simulink model "Preisach_1"  (R2015a)
settings: Solver=ode3  StartTime=0.0  StopTime=10.0  FixedStep=0.001  RelTol=1e-3
settings Model: Creator=spikelucky  LastModifiedBy=kr2112
settings DebuggingCC: UnderspecifiedInitializationDetection=Classic  MergeDetectMultiDrivingBlocksExec=none  SolverPrmCheckMsg=warning  StateNameClashWarn=warning

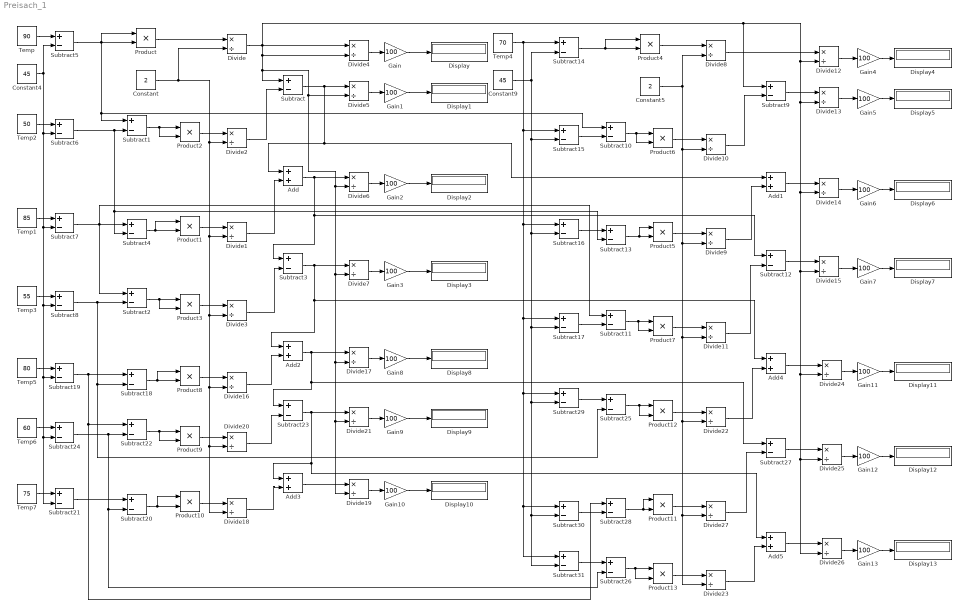
== system Preisach_1 ==
  Add{,1..5} (6 alike) : Sum
  Constant : Constant  Value=2
  Constant4 : Constant  Value=45
  Constant5 : Constant  Value=2
  Constant9 : Constant  Value=45
  Display{,1..13} (14 alike) : Display
  Divide{,1..27} (28 alike) : Product  Inputs=*/
  Gain{,1..13} (14 alike) : Gain  Gain=100
  Product{,1..13} (14 alike) : Product
  Subtract{,1..31} (32 alike) : Sum  Inputs=+-
  Temp : Constant  Value=90
  Temp1 : Constant  Value=85
  Temp2 : Constant  Value=50
  Temp3 : Constant  Value=55
  Temp4 : Constant  Value=70
  Temp5 : Constant  Value=80
  Temp6 : Constant  Value=60
  Temp7 : Constant  Value=75
  wires:
  Temp/1 -> Subtract5/1
  Product/1 -> Divide/1
  Product2/1 -> Divide2/1
  Divide2/1 -> Subtract/2
  Subtract1/1 -> Product2/2, Product2/1
  Product1/1 -> Divide1/1
  Divide1/1 -> Add/2
  Add/1 -> Divide6/1, Subtract3/1, Subtract12/1
  Product3/1 -> Divide3/1
  Subtract2/1 -> Product3/2, Product3/1
  Divide3/1 -> Subtract3/2
  Subtract4/1 -> Product1/2, Product1/1
  Divide4/1 -> Gain/1
  Gain/1 -> Display/1
  Gain1/1 -> Display1/1
  Divide5/1 -> Gain1/1
  Divide6/1 -> Gain2/1
  Gain2/1 -> Display2/1
  Divide7/1 -> Gain3/1
  Gain3/1 -> Display3/1
  Subtract3/1 -> Add4/1, Add2/1, Divide7/1
  Constant4/1 -> Subtract21/2, Subtract24/2, Subtract19/2, Subtract8/2, Subtract7/2, Subtract6/2, Subtract5/2
  Subtract5/1 -> Subtract10/1, Subtract1/1, Product/1, Product/2
  Subtract6/1 -> Subtract13/2, Subtract4/2, Subtract1/2
  Temp2/1 -> Subtract6/1
  Subtract7/1 -> Subtract2/1, Subtract11/1, Subtract4/1
  Temp1/1 -> Subtract7/1
  Subtract8/1 -> Subtract25/2, Subtract18/2, Subtract2/2
  Temp3/1 -> Subtract8/1
  Product4/1 -> Divide8/1
  Product6/1 -> Divide10/1
  Divide8/1 -> Divide12/1
  Divide10/1 -> Subtract9/2
  Subtract9/1 -> Divide13/1
  Subtract10/1 -> Product6/1, Product6/2
  Product5/1 -> Divide9/1
  Divide9/1 -> Add1/2
  Add1/1 -> Divide14/1
  Product7/1 -> Divide11/1
  Subtract11/1 -> Product7/2, Product7/1
  Divide11/1 -> Subtract12/2
  Subtract13/1 -> Product5/2, Product5/1
  Divide12/1 -> Gain4/1
  Gain4/1 -> Display4/1
  Gain5/1 -> Display5/1
  Divide13/1 -> Gain5/1
  Divide14/1 -> Gain6/1
  Gain6/1 -> Display6/1
  Divide15/1 -> Gain7/1
  Gain7/1 -> Display7/1
  Subtract12/1 -> Divide15/1
  Subtract14/1 -> Product4/1, Product4/2
  Subtract15/1 -> Subtract10/2
  Subtract16/1 -> Subtract13/1
  Subtract17/1 -> Subtract11/2
  Product8/1 -> Divide16/1
  Subtract18/1 -> Product8/2, Product8/1
  Subtract19/1 -> Subtract28/1, Subtract22/1, Subtract18/1
  Temp5/1 -> Subtract19/1
  Divide17/1 -> Gain8/1
  Gain8/1 -> Display8/1
  Divide16/1 -> Add2/2
  Product9/1 -> Divide20/1
  Subtract22/1 -> Product9/2, Product9/1
  Divide20/1 -> Subtract23/2
  Divide21/1 -> Gain9/1
  Gain9/1 -> Display9/1
  Subtract23/1 -> Add5/1, Add3/1, Divide21/1
  Subtract24/1 -> Subtract26/2, Subtract20/2, Subtract22/2
  Temp6/1 -> Subtract24/1
  Constant/1 -> Divide18/2, Divide20/2, Divide16/2, Divide3/2, Divide1/2, Divide2/2, Divide/2
  Product10/1 -> Divide18/1
  Subtract20/1 -> Product10/2, Product10/1
  Subtract21/1 -> Subtract20/1
  Temp7/1 -> Subtract21/1
  Divide19/1 -> Gain10/1
  Gain10/1 -> Display10/1
  Divide18/1 -> Add3/2
  Add3/1 -> Divide19/1
  Add2/1 -> Subtract23/1, Subtract27/1, Divide17/1
  Divide/1 -> Divide4/1, Subtract9/1, Divide12/2, Divide13/2, Divide14/2, Divide24/2, Divide26/2, Divide25/2, Divide15/2, Subtract/1, Divide7/2, Divide19/2, Divide21/2, Divide17/2, Divide6/2, Divide5/2, Divide4/2
  Temp4/1 -> Subtract17/1, Subtract30/1, Subtract31/1, Subtract29/1, Subtract16/1, Subtract15/1, Subtract14/1
  Product12/1 -> Divide22/1
  Divide22/1 -> Add4/2
  Add4/1 -> Divide24/1
  Subtract25/1 -> Product12/2, Product12/1
  Product11/1 -> Divide27/1
  Divide27/1 -> Subtract27/2
  Constant5/1 -> Divide10/2, Divide23/2, Divide27/2, Divide22/2, Divide11/2, Divide9/2, Divide8/2
  Product13/1 -> Divide23/1
  Subtract26/1 -> Product13/1, Product13/2
  Divide23/1 -> Add5/2
  Subtract28/1 -> Product11/2, Product11/1
  Divide24/1 -> Gain11/1
  Divide25/1 -> Gain12/1
  Gain12/1 -> Display12/1
  Divide26/1 -> Gain13/1
  Gain13/1 -> Display13/1
  Constant9/1 -> Subtract30/2, Subtract31/2, Subtract29/2, Subtract17/2, Subtract16/2, Subtract15/2, Subtract14/2
  Subtract29/1 -> Subtract25/1
  Subtract31/1 -> Subtract26/1
  Subtract27/1 -> Divide25/1
  Add5/1 -> Divide26/1
  Gain11/1 -> Display11/1
  Subtract30/1 -> Subtract28/2
  Subtract/1 -> Add/1, Add1/1, Divide5/1
